simulink subsystem "Motor"  (R2025a)
settings: Solver=VariableStepAuto  StartTime=0.0  StopTime=10.0  RelTol=1e-3
undefined symbols (not defined in the file): b, J, K, L, R
settings Model: Creator=JPIRES3  LastModifiedBy=JPIRES3

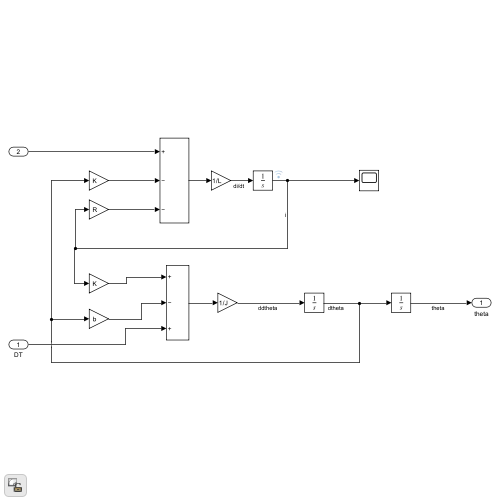
[thumbnail: Simulink's stored preview of the top-level diagram]
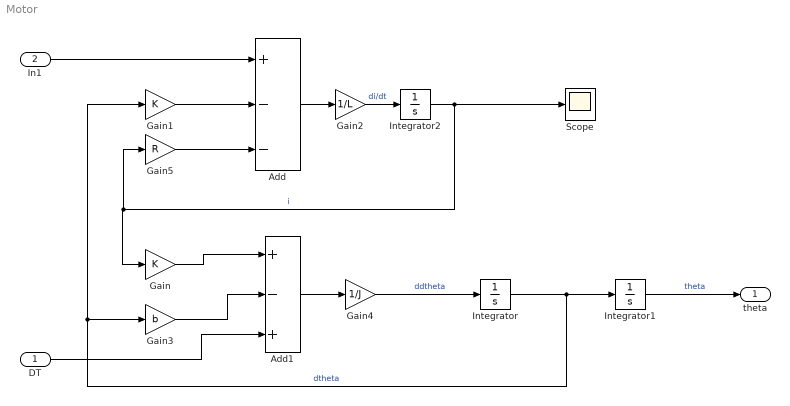
== system Motor ==
  DT : Inport
  In1 : Inport  Port=2
  Add : Sum  Inputs=+--
  Add1 : Sum  Inputs=+-+
  Gain : Gain  Gain=K
  Gain1 : Gain  Gain=K
  Gain2 : Gain  Gain=1/L
  Gain3 : Gain  Gain=b
  Gain4 : Gain  Gain=1/J
  Gain5 : Gain  Gain=R
  Integrator : Integrator
  Integrator1 : Integrator
  Integrator2 : Integrator
  Scope : Scope
      settings: ActiveDisplayYMinimum=-0.073405567669839467  ActiveDisplayYMaximum=0.031632687357691952
  theta : Outport
  wires:
  Integrator/1 -> Gain3/1, Gain1/1, Integrator1/1  "dtheta"
  Gain5/1 -> Add/3
  Add1/1 -> Gain4/1
  Gain1/1 -> Add/2
  Gain3/1 -> Add1/2
  Gain4/1 -> Integrator/1  "ddtheta"
  Gain/1 -> Add1/1
  Integrator2/1 -> Gain/1, Gain5/1, Scope/1  "i"
  Add/1 -> Gain2/1
  Gain2/1 -> Integrator2/1  "di/dt"
  Integrator1/1 -> theta/1  "theta"
  In1/1 -> Add/1
  DT/1 -> Add1/3
